simulink model "acmi5"  (Simulink 6.5)
settings: Solver=ode23t  StartTime=0.0  StopTime=7  RelTol=1e-3
undefined symbols (not defined in the file): powergui
libraries: powerlib x13, powerlib_extras x1
settings Model: Creator=RS  LastModifiedBy=RS

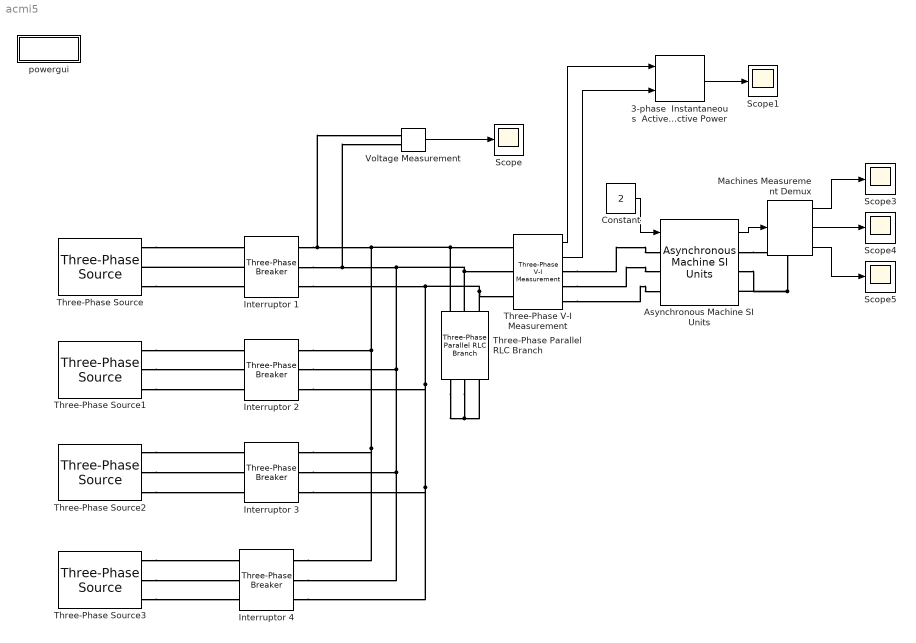
== system acmi5 ==
  3-phase  Instantaneous  Active & Reactive Power : powerlib_extras/Measurements/3-phase  Instantaneous  Active & Reactive Power  DialogController=PMDialogs.PMDefaultMaskDlg  SystemSampleTime=-1
  Asynchronous Machine SI Units : powerlib/Machines/Asynchronous Machine SI Units  DialogController=PMDialogs.PMDefaultMaskDlg  SystemSampleTime=-1  PresetModel=No  MechanicalLoad=Torque Tm  ShowDetailedParameters=on  RotorType=Wound  ReferenceFrame=Stationary  NominalParameters="[6.5*746    380    50]"  Stator="[0.63    0.00496]"  Rotor="[1.094    0.00496]"  Lm=0.105  Mechanical="[  0.3   0.01  2]"  PolePairs=2  InitialConditions="[ 1,0   0,0,0   0,0,0 ]"  Units=1  LoadFlowParameters=0  SimulateSaturation=off  Saturation=[9.9249,19.6672,38.0377,51.3988,69.2824,105.1337,152.5532,214.2421,303.1917;230, 322, 414, 460, 506, 552, 598, 644, 690]
  Constant : Constant  Value=2  OutDataType=sfix(16)  ConRadixGroup=Use specified scaling  OutScaling=2^0  SampleTime=inf  FramePeriod=inf
  Interruptor 1 : powerlib/Elements/Three-Phase Breaker  DialogController=PMDialogs.PMDefaultMaskDlg  SystemSampleTime=-1  InitialState=open  SwitchA=on  SwitchB=on  SwitchC=on  SwitchTimes="[0  0.4   3.8   4.2]"  External=off  BreakerResistance=0.001  SnubberResistance=1e6  SnubberCapacitance=inf  Measurements=None
  Interruptor 2 : powerlib/Elements/Three-Phase Breaker  DialogController=PMDialogs.PMDefaultMaskDlg  SystemSampleTime=-1  InitialState=open  SwitchA=on  SwitchB=on  SwitchC=on  SwitchTimes="[0.4   0.8    3.4   3.8]"  External=off  BreakerResistance=0.001  SnubberResistance=1e6  SnubberCapacitance=inf  Measurements=None
  Interruptor 3 : powerlib/Elements/Three-Phase Breaker  DialogController=PMDialogs.PMDefaultMaskDlg  SystemSampleTime=-1  InitialState=open  SwitchA=on  SwitchB=on  SwitchC=on  SwitchTimes="[0.81    1.2   3  3.4]"  External=off  BreakerResistance=0.001  SnubberResistance=1e6  SnubberCapacitance=inf  Measurements=None
  Interruptor 4 : powerlib/Elements/Three-Phase Breaker  DialogController=PMDialogs.PMDefaultMaskDlg  SystemSampleTime=-1  InitialState=open  SwitchA=on  SwitchB=on  SwitchC=on  SwitchTimes="[1.2   3]"  External=off  BreakerResistance=0.001  SnubberResistance=1e6  SnubberCapacitance=inf  Measurements=None
  Machines Measurement Demux : powerlib/Machines/Machines Measurement Demux  DialogController=PMDialogs.PMDefaultMaskDlg  SystemSampleTime=-1  machType=Asynchronous  ssm1=on  ssm2=on  ssm3=on  ssm4=on  ssm5=on  ssm6=on  sm1=off  sm2=off  sm3=off  sm4=off  sm5=off  sm6=off  sm7=off  sm8=on  sm9=off  sm10=off  sm11=off  sm115=off  sm12=off  sm13=off  sm14=off  asm1=off  asm2=off  asm3=off  asm4=off  asm5=on  asm6=off  asm7=off  asm8=off  asm9=on  asm10=on  asm11=off  pmsm1=on  pmsm2=on  pmsm3=on  pmsm4=off  pmsm5=on  pmsm6=on  pmsm7=on  lastType=1
  Scope{,1,3..5} (5 alike) : Scope
      Scope settings: MaxDataPoints=10000000  SampleInput=on  SampleTime=10e-6
      Scope1 settings: MaxDataPoints=10000000  SampleInput=on  SampleTime=10e-6
      Scope3 settings: SaveName=ScopeData3  MaxDataPoints=10000000  SampleInput=on  SampleTime=10e-6
      Scope4 settings: YMin=-165.791  YMax=-150.001  SaveName=ScopeData4  MaxDataPoints=10000000  SampleInput=on  SampleTime=10e-6
      Scope5 settings: SaveName=ScopeData5  MaxDataPoints=10000000  SampleInput=on  SampleTime=10e-6
  Three-Phase Parallel RLC Branch : powerlib/Elements/Three-Phase Parallel RLC Branch  Orientation=down  DialogController=PMDialogs.PMDefaultMaskDlg  PhysicalDomain=powersysdomain  SubClassName=unknown  LeftPortType=p1  RightPortType=p1  LConnTagsString=A|B|C  RConnTagsString=A|B|C  BranchType=R  Resistance=90000  Inductance=1e-3  Capacitance=1e-6  Measurements=None
  Three-Phase V-I Measurement : powerlib/Measurements/Three-Phase V-I Measurement  DialogController=PMDialogs.PMDefaultMaskDlg  SystemSampleTime=-1  VoltageMeasurement=phase-to-ground  SetLabelV=off  LabelV=Vabc  Vpu=off  CurrentMeasurement=yes  SetLabelI=off  LabelI=Iabc  Ipu=off  Pbase=100e6  Vbase=500e3  OutputType=Complex  PhasorSimulation=off  PSBequivalent=0
  Three-Phase Source : powerlib/Electrical Sources/Three-Phase Source  DialogController=PMDialogs.PMDefaultMaskDlg  SystemSampleTime=-1  Voltage=380*1/4  PhaseAngle=0  Frequency=50*1/4  InternalConnection=Yg  SpecifyImpedance=off  Resistance=0.0001  Inductance=0.00001  ShortCircuitLevel=100e6  BaseVoltage=25e3  XRratio=7
  Three-Phase Source1 : powerlib/Electrical Sources/Three-Phase Source  DialogController=PMDialogs.PMDefaultMaskDlg  SystemSampleTime=-1  Voltage=380*1/2  PhaseAngle=0  Frequency=50*1/2  InternalConnection=Yg  SpecifyImpedance=off  Resistance=0.0001  Inductance=0.00001  ShortCircuitLevel=100e6  BaseVoltage=25e3  XRratio=7
  Three-Phase Source2 : powerlib/Electrical Sources/Three-Phase Source  DialogController=PMDialogs.PMDefaultMaskDlg  SystemSampleTime=-1  Voltage=380*3/4  PhaseAngle=0  Frequency=50*3/4  InternalConnection=Yg  SpecifyImpedance=off  Resistance=0.0001  Inductance=0.00001  ShortCircuitLevel=100e6  BaseVoltage=25e3  XRratio=7
  Three-Phase Source3 : powerlib/Electrical Sources/Three-Phase Source  DialogController=PMDialogs.PMDefaultMaskDlg  SystemSampleTime=-1  Voltage=380  PhaseAngle=0  Frequency=50  InternalConnection=Yg  SpecifyImpedance=off  Resistance=0.0001  Inductance=0.00001  ShortCircuitLevel=100e6  BaseVoltage=25e3  XRratio=7
  Voltage Measurement : powerlib/Measurements/Voltage Measurement  DialogController=PMDialogs.PMDefaultMaskDlg  SystemSampleTime=-1  PhasorSimulation=off  OutputType=Complex  PSBequivalent=0
  powergui : Subsystem  AncestorBlock=powerlib/powergui  InitFcn=powergui( 'InitFcn_Callback' , gcb , 0 , [ ] );  mask(PSB option menu block){SimulationMode=Continuous, SampleTime=50e-6, echomessages=off, RestoreLinks=warning, x0status=blocks, Frange=[0:2:500], Ylog=off, Xlog=on, ShowGrid=off, save=off, variable=ZData, structure=, ZoomFFT=on, StartTime=0.0, cycles=1, DisplayStyle=1, fundamental=60, FreqAxis=off, MaxFrequency=1000, frequencyindice=50, frequencyindicesteady=1, RmsSteady=1, display=off, Ts=0, frequency=60, methode=off, HookPort=off, Interpol=off}
      mask prompts: SimulationMode "Simulation mode"; SampleTime "Sample time Ts (when simulation mode is Discrete) (s)"; echomessages "Echo  Messages"; RestoreLinks "Restore disabled links"; x0status "Initial electrical states status"; Frange "Impedance tool: Frequency Range"; Ylog "Impedance tool: Log impedance"; Xlog "Impedance tool: log Frequency"; ShowGrid "Impedance tool: grid"; save "Impedance tool: Save Data To Workspace"; variable "Impedance tool: Variable Name"; structure "Structure Name (PSBFFTSCOPE)"; ZoomFFT "ZoomFFT (PSBFFTSCOPE)"; StartTime "Start Time (PSBFFTSCOPE)"; cycles "Cycles (PSBFFTSCOPE)"; DisplayStyle "Display style (PSBFFTSCOPE)"; fundamental "Fundamental (PSBFFTSCOPE)"; FreqAxis "Frequency Axis (PSBFFTSCOPE)"; MaxFrequency "Max Frequency (PSBFFTSCOPE)"; frequencyindice "Load flow frequency (Hz)"; frequencyindicesteady "Frequency indice (STEADYSTATE)"; RmsSteady "RMS display (STEADYSTATE)"; display "Display Results"; Ts "OBSOLETE 1"; frequency "Phasor frequency (Hz)"; methode "Phasor simulation"; HookPort "Hook port"; Interpol "Interpolate"
      mask init:
      | powerlibroot = which('powersysdomain');
      | PSBroot = powerlibroot(1:end-16);
      | %
      | switch SimulationMode
      | 	case 1
      | 		message=sprintf('Continuous');
      | 	case 2
      |         SampleTimeeval=evalin('base',SampleTime,'NaN');
      |         if isnan(SampleTimeeval)
      |             message=sprintf('Warning !!,\nUndefined sample time');
      |         else
      |             message=sprintf('Discrete,\nTs = %.4g s.',SampleTimeeval);
      |         end
      | 	case 3
      | 		message=sprintf('Phasors');
      | end
      | if strcmp(bdroot,'powerlib')
      |   message='powergui';
      | end
      | power_initmask();
      settings: CopyFcn=powergui( 'Copy_Callback' , gcb , 0 , [ ] );  ModelCloseFcn=powergui( 'CloseButton_Callback' , gcb , [ ] , [ ] );  PreSaveFcn=powergui( 'CloseButton_Callback' , gcb , [ ] , [ ] );  NameChangeFcn=powergui( 'NameChangeFcn_Callback' , gcb , 0 , [ ] );
      settings: DeleteFcn=|
      | powergui( 'Copy_Callback' , gcb , 1 , [ ] );
      | powergui( 'CloseButton_Callback' , gcb , [ ] , [ ] );
      settings: OpenFcn=|
      | if (power_openblockproxy ('secondary'))
      | powergui(gcb,'PM')
      | end;
      mask Help: web(psbhelp)
      mask StyleString: popup(Continuous|Discrete|Phasor),edit,checkbox,popup(yes|warning|no),popup(blocks|steady|zero),edit,checkbox,checkbox,checkbox,checkbox,edit,edit,checkbox,edit,edit,edit,edit,checkbox,edit,edit,edit,edit,checkbox,edit,edit,checkbox,checkbox,checkbox
      mask CallbackString: ||||||||||||||||||||||||||powergui('HookPort',[],[],gcb);|
      mask Display: disp(message)
  wires:
  Constant/1 -> Asynchronous Machine SI Units/1
  Asynchronous Machine SI Units/1 -> Machines Measurement Demux/1
  Machines Measurement Demux/2 -> Scope4/1
  Machines Measurement Demux/1 -> Scope3/1
  Machines Measurement Demux/3 -> Scope5/1
  Voltage Measurement/1 -> Scope/1
  Three-Phase V-I Measurement/1 -> 3-phase  Instantaneous  Active & Reactive Power/1
  Three-Phase V-I Measurement/2 -> 3-phase  Instantaneous  Active & Reactive Power/2
  3-phase  Instantaneous  Active & Reactive Power/1 -> Scope1/1
  connections:
  Three-Phase Source/RConn1 -- Interruptor 1/LConn1
  Interruptor 1/LConn2 -- Three-Phase Source/RConn2
  Asynchronous Machine SI Units/RConn1 -- Asynchronous Machine SI Units/RConn3 -- Asynchronous Machine SI Units/RConn2
  Three-Phase Source/RConn3 -- Interruptor 1/LConn3
  Three-Phase Source1/RConn1 -- Interruptor 2/LConn1
  Three-Phase Source1/RConn2 -- Interruptor 2/LConn2
  Three-Phase Source1/RConn3 -- Interruptor 2/LConn3
  Three-Phase Source2/RConn1 -- Interruptor 3/LConn1
  Three-Phase Source2/RConn2 -- Interruptor 3/LConn2
  Three-Phase Source2/RConn3 -- Interruptor 3/LConn3
  Three-Phase Source3/RConn1 -- Interruptor 4/LConn1
  Three-Phase Source3/RConn2 -- Interruptor 4/LConn2
  Three-Phase Source3/RConn3 -- Interruptor 4/LConn3
  Three-Phase Parallel RLC Branch/LConn1 -- Interruptor 2/RConn1 -- Interruptor 4/RConn1 -- Interruptor 3/RConn1 -- Interruptor 1/RConn1 -- Voltage Measurement/LConn1 -- Three-Phase V-I Measurement/LConn1
  Three-Phase Parallel RLC Branch/LConn2 -- Interruptor 2/RConn2 -- Interruptor 4/RConn2 -- Interruptor 3/RConn2 -- Interruptor 1/RConn2 -- Voltage Measurement/LConn2 -- Three-Phase V-I Measurement/LConn2
  Three-Phase Parallel RLC Branch/LConn3 -- Interruptor 1/RConn3 -- Interruptor 2/RConn3 -- Interruptor 4/RConn3 -- Interruptor 3/RConn3 -- Three-Phase V-I Measurement/LConn3
  Three-Phase Parallel RLC Branch/RConn1 -- Three-Phase Parallel RLC Branch/RConn3 -- Three-Phase Parallel RLC Branch/RConn2
  Three-Phase V-I Measurement/RConn1 -- Asynchronous Machine SI Units/LConn1
  Three-Phase V-I Measurement/RConn2 -- Asynchronous Machine SI Units/LConn2
  Three-Phase V-I Measurement/RConn3 -- Asynchronous Machine SI Units/LConn3

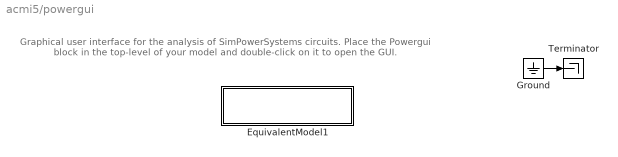
== system acmi5/powergui ==
  note: Graphical user interface for the analysis of  SimPowerSystems circuits.
      | Place the Powergui block in the top-level of your model and double-click
      | on it to open the GUI.
  EquivalentModel1 : Subsystem
      mask init:
      | SPS = get_param(gcbh,'UserData');
      | if isempty(SPS)
      |     A=0;
      |     B=0;
      |     C=0;
      |     D=0;
      |     x0=0;
      |     SwitchResistance=1;
      |     SwitchType=1;
      |     SwitchGateInitialValue=1;
      |     OutputsToResetToZero=1;
      | else
      | 	A=SPS.A;
      |     B=SPS.B;
      |     C=SPS.C;
      |     D=SPS.D;
      |     x0=SPS.x0;
      |     SwitchResistance=SPS.SwitchResistance;
      |     SwitchType=SPS.SwitchType;
      |     SwitchGateInitialValue=SPS.SwitchGateInitialValue;
      |     OutputsToResetToZero=SPS.YSwitchCurrent;
      | end
      mask Display:
      | color('blue')
      | disp('EQUIVALENT CIRCUIT')
  Ground : Ground
  Terminator : Terminator
  wires:
  Ground/1 -> Terminator/1

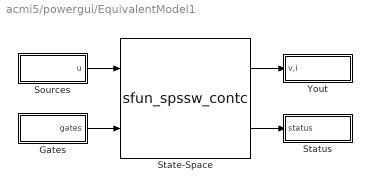
== system acmi5/powergui/EquivalentModel1 ==
  Gates : Subsystem
  Sources : Subsystem
  State-Space : S-Function  FunctionName=sfun_spssw_contc  Parameters=A, B, C, D, x0, SwitchResistance ,SwitchType, SwitchGateInitialValue, OutputsToResetToZero
  Status : Subsystem
  Yout : Subsystem
  wires:
  Gates/1(gates) -> State-Space/2
  Sources/1(u) -> State-Space/1
  State-Space/2 -> Status/1(status)
  State-Space/1 -> Yout/1(v,i)

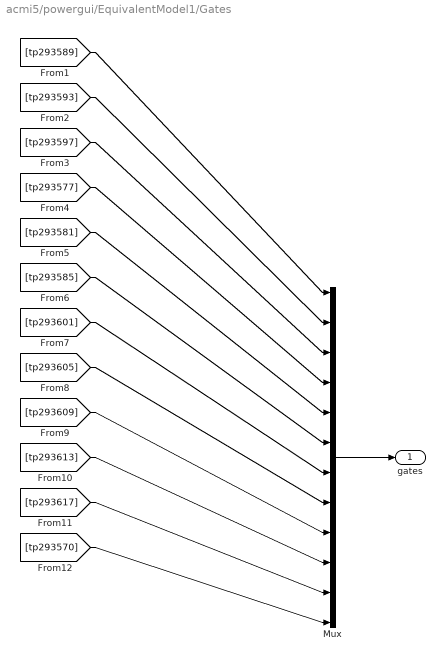
== system acmi5/powergui/EquivalentModel1/Gates ==
  Mux : Mux  Inputs=[1 1 1 1 1 1 1 1 1 1 1 1]
  gates : Outport
  wires:
  Mux/1 -> gates/1
  [tp293589] -> Mux/1
  [tp293593] -> Mux/2
  [tp293597] -> Mux/3
  [tp293577] -> Mux/4
  [tp293581] -> Mux/5
  [tp293585] -> Mux/6
  [tp293601] -> Mux/7
  [tp293605] -> Mux/8
  [tp293609] -> Mux/9
  [tp293613] -> Mux/10
  [tp293617] -> Mux/11
  [tp293570] -> Mux/12

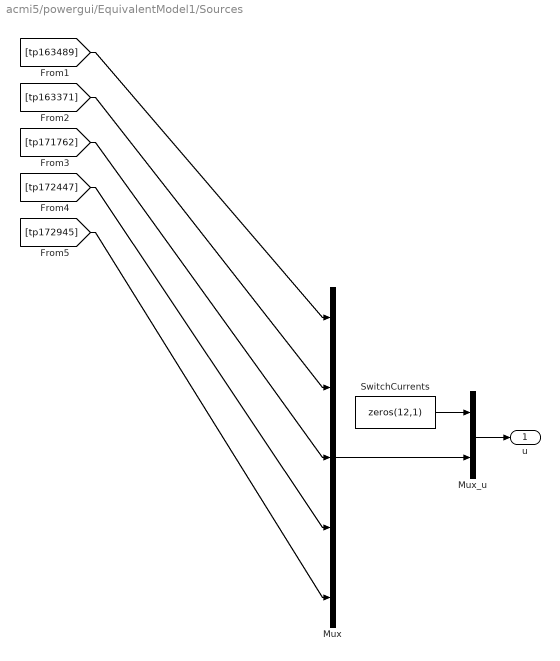
== system acmi5/powergui/EquivalentModel1/Sources ==
  Mux : Mux  Inputs=[4 3 3 3 3]
  Mux_u : Mux  Inputs=[12 16]
  SwitchCurrents : Constant  Value=zeros(12,1)  OutDataType=sfix(16)  ConRadixGroup=Use specified scaling  OutScaling=2^0  SampleTime=inf  FramePeriod=inf
  u : Outport
  wires:
  Mux/1 -> Mux_u/2
  SwitchCurrents/1 -> Mux_u/1
  Mux_u/1 -> u/1
  [tp163489] -> Mux/1
  [tp163371] -> Mux/2
  [tp171762] -> Mux/3
  [tp172447] -> Mux/4
  [tp172945] -> Mux/5

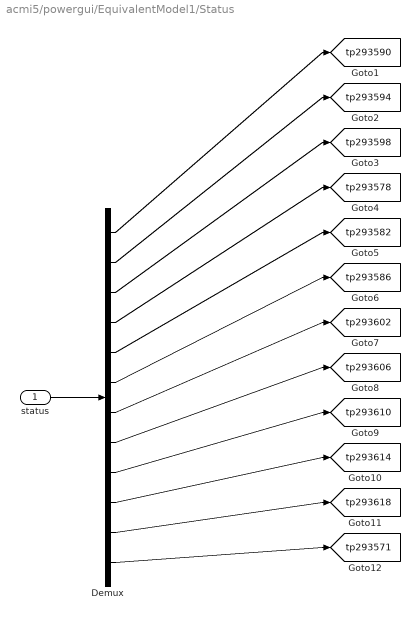
== system acmi5/powergui/EquivalentModel1/Status ==
  status : Inport
  Demux : Demux  Outputs=[1 1 1 1 1 1 1 1 1 1 1 1]
  tag scope: tp293571=global, tp293578=global, tp293582=global, tp293586=global, tp293590=global, tp293594=global, tp293598=global, tp293602=global, tp293606=global, tp293610=global, tp293614=global, tp293618=global
  wires:
  status/1 -> Demux/1
  Demux/1 -> [tp293590]
  Demux/2 -> [tp293594]
  Demux/3 -> [tp293598]
  Demux/4 -> [tp293578]
  Demux/5 -> [tp293582]
  Demux/6 -> [tp293586]
  Demux/7 -> [tp293602]
  Demux/8 -> [tp293606]
  Demux/9 -> [tp293610]
  Demux/10 -> [tp293614]
  Demux/11 -> [tp293618]
  Demux/12 -> [tp293571]

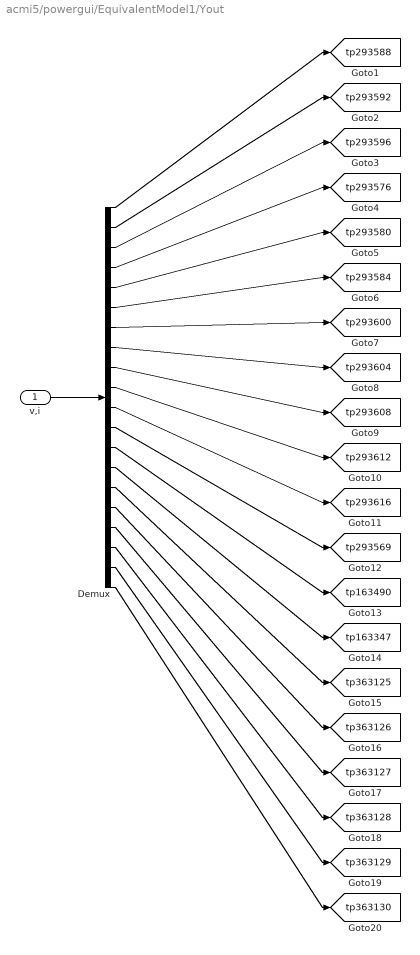
== system acmi5/powergui/EquivalentModel1/Yout ==
  v,i : Inport
  Demux : Demux  Outputs=[1 1 1 1 1 1 1 1 1 1 1 1 4 1 1 1 1 1 1 1]
  tag scope: tp163347=global, tp163490=global, tp293569=global, tp293576=global, tp293580=global, tp293584=global, tp293588=global, tp293592=global, tp293596=global, tp293600=global, tp293604=global, tp293608=global, tp293612=global, tp293616=global, tp363125=global, tp363126=global, tp363127=global, tp363128=global, tp363129=global, tp363130=global
  wires:
  v,i/1 -> Demux/1
  Demux/1 -> [tp293588]
  Demux/2 -> [tp293592]
  Demux/3 -> [tp293596]
  Demux/4 -> [tp293576]
  Demux/5 -> [tp293580]
  Demux/6 -> [tp293584]
  Demux/7 -> [tp293600]
  Demux/8 -> [tp293604]
  Demux/9 -> [tp293608]
  Demux/10 -> [tp293612]
  Demux/11 -> [tp293616]
  Demux/12 -> [tp293569]
  Demux/13 -> [tp163490]
  Demux/14 -> [tp163347]
  Demux/15 -> [tp363125]
  Demux/16 -> [tp363126]
  Demux/17 -> [tp363127]
  Demux/18 -> [tp363128]
  Demux/19 -> [tp363129]
  Demux/20 -> [tp363130]
